simulink model "euler"  (R2020a)
settings: Solver=VariableStepAuto  StartTime=0.0  StopTime=10.0  RelTol=1e-3
settings Model: Creator=surya  LastModifiedBy=surya

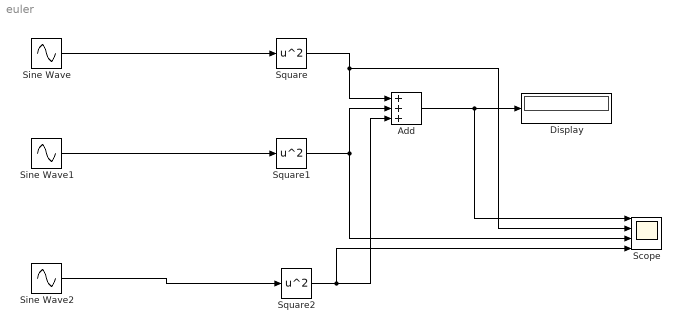
== system euler ==
  Add : Sum  Inputs=+++
  Display : Display
  Scope : Scope  NumInputPorts=4
  Sine Wave : Sin  Amplitude=100  Frequency=50  SampleTime=0
  Sine Wave1 : Sin  Amplitude=100  Frequency=50  Phase=120  SampleTime=0
  Sine Wave2 : Sin  Amplitude=100  Frequency=50  Phase=240  SampleTime=0
  Square : Math  Operator=square  SaturateOnIntegerOverflow=on
  Square1 : Math  Operator=square  SaturateOnIntegerOverflow=on
  Square2 : Math  Operator=square  SaturateOnIntegerOverflow=on
  wires:
  Sine Wave/1 -> Square/1
  Sine Wave1/1 -> Square1/1
  Square1/1 -> Add/2, Scope/3
  Square/1 -> Add/1, Scope/2
  Add/1 -> Scope/1, Display/1
  Sine Wave2/1 -> Square2/1
  Square2/1 -> Scope/4, Add/3
